simulink model "lab1_closedLoop_model"  (R2020b)
settings: Solver=VariableStepAuto  StartTime=0.0  StopTime=10.0  RelTol=1e-3
values from neighbouring files (symbols this model uses):
  DCmotor =     [DCmotor.mat]
undefined symbols (not defined in the file or in its folder): clock_c
libraries: simulink x2
settings Model: Creator=MSI  LastModifiedBy=MSI

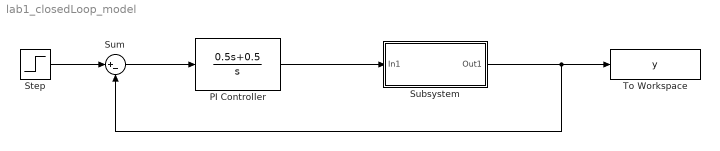
== system lab1_closedLoop_model ==
  PI Controller : TransferFcn  Numerator=[0.5 0.5]  Denominator=[1 0]
  Step : Step  Time=0  After=120  SampleTime=0
  Subsystem : Subsystem
  Sum : Sum  Inputs=|+-
  To Workspace : ToWorkspace  VariableName=y  SaveFormat=Timeseries  SampleTime=-1
  wires:
  Step/1 -> Sum/1
  PI Controller/1 -> Subsystem/1(In1)
  Subsystem/1(Out1) -> Sum/2, To Workspace/1
  Sum/1 -> PI Controller/1

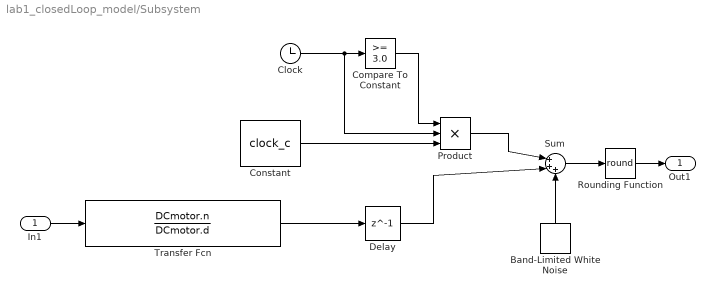
== system lab1_closedLoop_model/Subsystem ==
  In1 : Inport
  Band-Limited White Noise : simulink/Sources/Band-Limited White Noise  Cov=[0.005]  Ts=0.01  seed=[23341]
  Clock : Clock
  Compare To Constant : simulink/Logic and Bit Operations/Compare To Constant  relop=>=  const=3.0  OutDataTypeStr=uint8
  Constant : Constant  Value=clock_c
  Delay : Delay  DelayLength=1
  Product : Product  Inputs=3
  Rounding Function : Rounding  Operator=round
  Sum : Sum  Inputs=|+++
  Transfer Fcn : TransferFcn  Numerator=DCmotor.n  Denominator=DCmotor.d
  Out1 : Outport
  wires:
  Compare To Constant/1 -> Product/1
  Product/1 -> Sum/1
  In1/1 -> Transfer Fcn/1
  Clock/1 -> Product/2, Compare To Constant/1
  Sum/1 -> Rounding Function/1
  Constant/1 -> Product/3
  Delay/1 -> Sum/2
  Band-Limited White Noise/1 -> Sum/3
  Rounding Function/1 -> Out1/1
  Transfer Fcn/1 -> Delay/1
